simulink model "needle2"  (R2015a)
settings: Solver=ode4  StartTime=0.0  StopTime=100  FixedStep=0.001  RelTol=1e-3
settings Model: Creator=LAB425  LastModifiedBy=LAB425

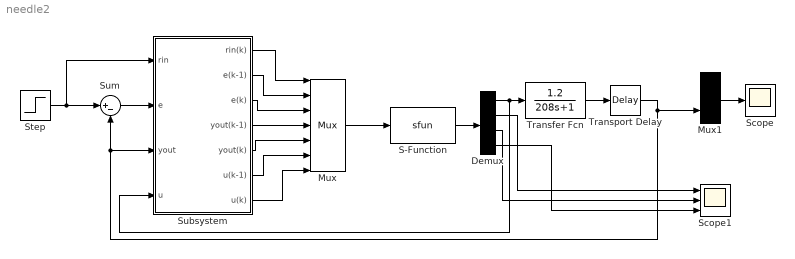
== system needle2 ==
  Demux : Demux
  Mux : Mux  Inputs=7
  Mux1 : Mux  Inputs=2
  S-Function : S-Function  FunctionName=sfun
  Scope : Scope
  Scope1 : Scope  NumInputPorts=3
      settings: YMin=-5~-5~-5  YMax=5~5~5
  Step : Step  SampleTime=0
  Subsystem : Subsystem
  Sum : Sum  Inputs=|+-
  Transfer Fcn : TransferFcn  Numerator=[1.2]  Denominator=[208 1]
  Transport Delay : TransportDelay  DelayTime=0
  wires:
  Mux/1 -> S-Function/1
  Subsystem/1(rin(k)) -> Mux/1
  Subsystem/2(e(k-1)) -> Mux/2
  Subsystem/3(e(k)) -> Mux/3
  Subsystem/4(yout(k-1)) -> Mux/4
  Subsystem/5(yout(k)) -> Mux/5
  Subsystem/6(u(k-1)) -> Mux/6
  Subsystem/7(u(k)) -> Mux/7
  Sum/1 -> Subsystem/2(e)
  Step/1 -> Subsystem/1(rin), Sum/1
  S-Function/1 -> Demux/1
  Demux/1 -> Subsystem/4(u), Transfer Fcn/1
  Transfer Fcn/1 -> Transport Delay/1
  Transport Delay/1 -> Mux1/2, Subsystem/3(yout), Sum/2
  Demux/2 -> Scope1/1
  Demux/3 -> Scope1/2
  Demux/4 -> Scope1/3
  Mux1/1 -> Scope/1

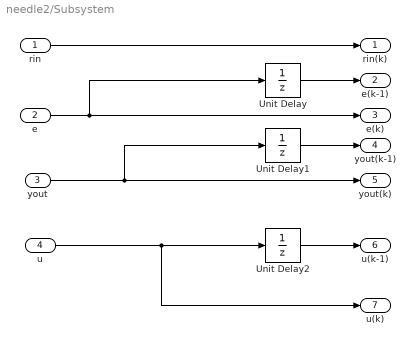
== system needle2/Subsystem ==
  rin : Inport
  e : Inport  Port=2
  yout : Inport  Port=3
  u : Inport  Port=4
  Unit Delay : UnitDelay  SampleTime=-1
  Unit Delay1 : UnitDelay  SampleTime=-1
  Unit Delay2 : UnitDelay  SampleTime=-1
  rin(k) : Outport
  e(k-1) : Outport  Port=2
  e(k) : Outport  Port=3
  yout(k-1) : Outport  Port=4
  yout(k) : Outport  Port=5
  u(k-1) : Outport  Port=6
  u(k) : Outport  Port=7
  wires:
  rin/1 -> rin(k)/1
  Unit Delay/1 -> e(k-1)/1
  Unit Delay1/1 -> yout(k-1)/1
  Unit Delay2/1 -> u(k-1)/1
  e/1 -> e(k)/1, Unit Delay/1
  yout/1 -> yout(k)/1, Unit Delay1/1
  u/1 -> u(k)/1, Unit Delay2/1
